simulink library "PV_lib"  (R2016b)
settings: Solver=ode45  StartTime=0.0  StopTime=10.0  RelTol=1e-3  EnableMultiTasking=on
undefined symbols (not defined in the file): C, D, DiscIntNeverNeededParam, f, I_ki, I_kp, Iac_max, Id_at_max, Iq_at_max, L, PLL_Ki, PLL_Kp, PLL_time_step, Roff, Tau, Td_es_min, Tds, Ts, Vdc_max
libraries: powerlib x42, simulink x16, cstextras x4, powerlib_extras x3, Batt_lib x1, powerlib_meascontrol x1
(part 2 of 2)

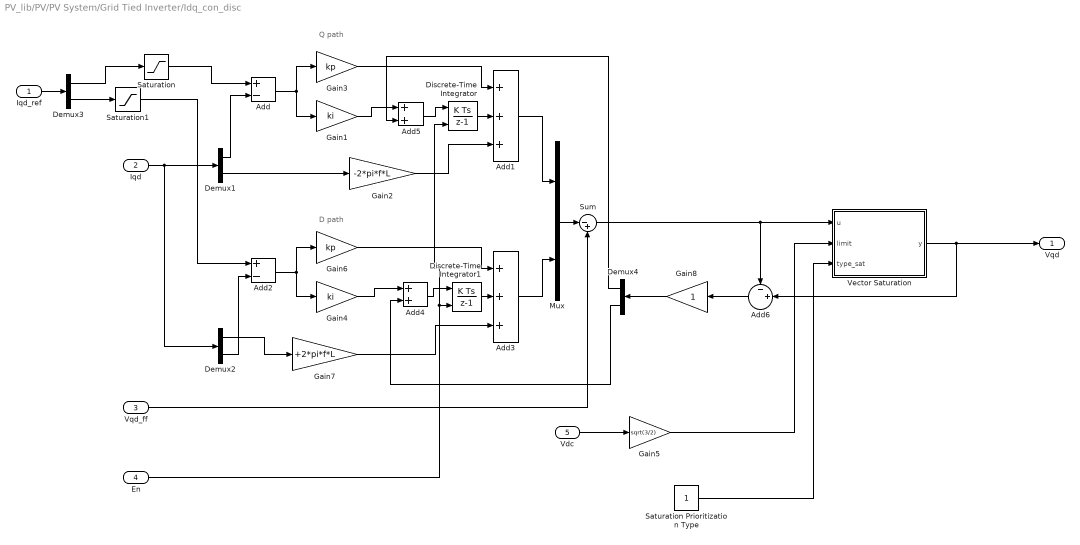
== system PV_lib/PV/PV System/Grid Tied Inverter/Idq_con_disc ==
  note: D path
  note: Q path
  Iqd_ref : Inport
  Iqd : Inport  Port=2
  Vqd_ff : Inport  Port=3  PortDimensions=2
  En : Inport  Port=4  OutDataTypeStr=boolean  PortDimensions=1
  Vdc : Inport  Port=5  PortDimensions=1
  Add : Sum  Inputs=+-
  Add1 : Sum  Inputs=+++
  Add2 : Sum  Inputs=+-
  Add3 : Sum  Inputs=+++
  Add4 : Sum
  Add5 : Sum
  Add6 : Sum  Inputs=-+|
  Demux{1..4} (4 alike) : Demux  Outputs=2
  Discrete-Time Integrator : DiscreteIntegrator  ExternalReset=rising  InitialConditionSetting=Compatibility  SampleTime=Ts  ICPrevOutput=DiscIntNeverNeededParam  ICPrevScaledInput=DiscIntNeverNeededParam
  Discrete-Time Integrator1 : DiscreteIntegrator  ExternalReset=rising  InitialConditionSetting=Compatibility  SampleTime=Ts  ICPrevOutput=DiscIntNeverNeededParam  ICPrevScaledInput=DiscIntNeverNeededParam
  Gain1 : Gain  Gain=ki
  Gain2 : Gain  Gain=-2*pi*f*L
  Gain3 : Gain  Gain=kp
  Gain4 : Gain  Gain=ki
  Gain5 : Gain  Gain=sqrt(3/2)
  Gain6 : Gain  Gain=kp
  Gain7 : Gain  Gain=+2*pi*f*L
  Gain8 : Gain
  Mux : Mux  Inputs=2
  Saturation : Saturate  UpperLimit=iq_max  LowerLimit=-iq_max
  Saturation Prioritization Type : Constant
  Saturation1 : Saturate  UpperLimit=id_max  LowerLimit=-id_max
  Sum : Sum  Inputs=|-+
  Vector Saturation : MATLAB Function  TreatAsAtomicUnit=on
  Vqd : Outport
  wires:
  Vdc/1 -> Gain5/1
  Add6/1 -> Gain8/1
  Gain5/1 -> Vector Saturation/2(limit)
  Saturation Prioritization Type/1 -> Vector Saturation/3(type_sat)
  Vqd_ff/1 -> Sum/2
  Demux2/1 -> Gain7/1
  Demux4/1 -> Add5/2
  Saturation/1 -> Add/1
  Saturation1/1 -> Add2/1
  Iqd_ref/1 -> Demux3/1
  Gain8/1 -> Demux4/1
  Add2/1 -> Gain6/1, Gain4/1
  Demux1/2 -> Gain2/1
  Vector Saturation/1(y) -> Add6/2, Vqd/1
  Demux1/1 -> Add/2
  Gain3/1 -> Add1/1
  Sum/1 -> Add6/1, Vector Saturation/1(u)
  Add1/1 -> Mux/1
  Gain4/1 -> Add4/1
  Add5/1 -> Discrete-Time Integrator/1
  Demux3/1 -> Saturation/1
  Add4/1 -> Discrete-Time Integrator1/1
  Iqd/1 -> Demux1/1, Demux2/1
  Discrete-Time Integrator/1 -> Add1/2
  Demux3/2 -> Saturation1/1
  Gain2/1 -> Add1/3
  Gain1/1 -> Add5/1
  En/1 -> Discrete-Time Integrator1/2, Discrete-Time Integrator/2
  Add3/1 -> Mux/2
  Demux2/2 -> Add2/2
  Gain7/1 -> Add3/3
  Discrete-Time Integrator1/1 -> Add3/2
  Mux/1 -> Sum/1
  Demux4/2 -> Add4/2
  Gain6/1 -> Add3/1
  Add/1 -> Gain3/1, Gain1/1

== system PV_lib/PV/PV System/Grid Tied Inverter/Modulator ==
  Vqd : Inport
  Vdc : Inport  Port=2
  Delay : Delay  DelayLength=1  InitialCondition=[0 0]  SampleTime=Ts
  IC : InitialCondition  Value=Vdc_nom
  Mult1 : Product  Inputs=*/
  Saturation : Saturate  UpperLimit=1  LowerLimit=-1
  dqd : Outport
  wires:
  Mult1/1 -> Saturation/1
  Saturation/1 -> Delay/1
  Vqd/1 -> Mult1/1
  Vdc/1 -> IC/1
  IC/1 -> Mult1/2
  Delay/1 -> dqd/1

== system PV_lib/PV/PV System/Grid Tied Inverter/PLL_disc ==
  note: Theta = 0 at phase A start.
  note: This block should use a normalized to +-1 abc input voltage
  abc : Inport  PortDimensions=3
  Demux1 : Demux  Outputs=2
  Discrete VCO : Subsystem
  Interval Test : simulink/Logic and Bit Operations/Interval Test  IntervalClosedRight=on  uplimit=PLL_lock_window  IntervalClosedLeft=on  lowlimit=-PLL_lock_window  OutDataTypeStr=boolean
  Interval Test1 : simulink/Logic and Bit Operations/Interval Test  IntervalClosedRight=on  uplimit=2*pi*f*(1+PLL_freq_range)  IntervalClosedLeft=on  lowlimit=2*pi*f*(1-PLL_freq_range)  OutDataTypeStr=boolean
  LTI System : Subsystem  BlockChoice=CSS  mask(LTI Block){sys=c2d(tf(1,[1/(f*2*2*pi),1]),Ts), IC=[]}
      mask prompts: sys "LTI system variable"; IC "Initial states (state-space only)"
      mask help:
      | The LTI System block accepts both continuous and discrete LTI models as defined in the Control System Toolbox. Transfer function, state-space, and zero-pole-gain formats are all supported in this block.
      |
      | Note: Initial states are only meaningful for state-space systems.
      mask init:
      | try
      |    % read data to initialize mask variables
      |    [D,Ts,Tdi,Tdo,Tdio,x0,sysname]=...
      |       ltimask('Initialize',gcb,sys,IC);
      |    % update contents
      |    model = bdroot;
      |    df = get_param(model,'dirty');
      |    ltimask('UpdateDiagram',gcb,D,Ts,Tdio);
      |    try      
      |       % Attempt to modify locked library -> error
      |       % Makes block show ??? when loading CSTBLOCKS
      |       % for the first time
      |       set_param(model,'dirty',df)
      |    end
      | catch ME
      |    sys = [];  IC = [];   sysname = '???';
      |    throw(ME)
      | end
      mask Help:
      | The LTI System block accepts any of the three standard LTI models described in the Control System Toolbox: transfer function, zero/pole/gain, or state space. Internally, LTI models will be converted to their state space equivalent for evaluation.
      | <p>
      | In the editable text box labeled <b>LTI System Variable</b>, enter a valid LTI model.
      | <p>
      | In the editable text box labeled <b>Initial States</b> enter the initial state vector.  Initial states are only valid for state-space systems.
      | <p>
      | See also TF, ZPK, SS, LTIMODELS.
      mask Callback sys: ltimask('MaskLTICallback',gcb);
      mask Display: disp(sysname)
  Logical Operator : Logic  AllPortsSameDT=off  OutDataTypeStr=boolean
  PID Controller : simulink/Continuous/PID Controller  Controller=PID  TimeDomain=Discrete-time  SampleTime=Ts  IntegratorMethod=Forward Euler  FilterMethod=Forward Euler  Form=Parallel  UseFilter=on  ControllerParametersSource=internal  P=PLL_Kp  I=PLL_Ki  D=0  N=100  InitialConditionSource=internal  InitialConditionForIntegrator=2*pi*f  InitialConditionForFilter=0  ExternalReset=none  ZeroCross=off  LimitOutput=on  UpperSaturationLimit=2*pi*(f*(1+PLL_freq_range))  LowerSaturationLimit=2*pi*(f*(1-PLL_freq_range))  LinearizeAsGain=on  AntiWindupMode=clamping  Kb=1  TrackingMode=off  Kt=1  PParamMin=[]  PParamMax=[]  IParamMin=[]  IParamMax=[]  DParamMin=[]  DParamMax=[]  NParamMin=[]  NParamMax=[]  KbParamMin=[]  KbParamMax=[]  KtParamMin=[]  KtParamMax=[]  POutMin=[]  POutMax=[]  IOutMin=[]  IOutMax=[]  DOutMin=[]  DOutMax=[]  NOutMin=[]  NOutMax=[]  KbOutMin=[]  KbOutMax=[]  KtOutMin=[]  KtOutMax=[]  IntegratorOutMin=[]  IntegratorOutMax=[]  FilterOutMin=[]  FilterOutMax=[]  SumOutMin=[]  SumOutMax=[]  SumI1OutMin=[]  SumI1OutMax=[]  SumI2OutMin=[]  SumI2OutMax=[]  SumI3OutMin=[]  SumI3OutMax=[]  SumDOutMin=[]  SumDOutMax=[]  SaturationOutMin=[]  SaturationOutMax=[]  IntegratorContinuousStateAttributes=''  IntegratorStateMustResolveToSignalObject=off  IntegratorRTWStateStorageClass=Auto  FilterContinuousStateAttributes=''  FilterStateMustResolveToSignalObject=off  FilterRTWStateStorageClass=Auto  DifferentiatorICPrevScaledInput=0  DifferentiatorOutMin=[]  DifferentiatorOutMax=[]
  Rate Transition : RateTransition  OutPortSampleTime=PLL_time_step
  Subsystem : Subsystem
  Sum : Sum  Inputs=|+-
  Terminator : Terminator
  Terminator1 : Terminator
  Terminator2 : Terminator
  zero : Constant  Value=0
  theta : Outport
  freq : Outport  Port=2
  locked : Outport  Port=3
  wires:
  PID Controller/1 -> freq/1, Discrete VCO/1(In1), Interval Test1/1
  LTI System/1(Out1) -> Interval Test/1
  Demux1/2 -> Terminator2/1  "Vq"
  Demux1/1 -> Sum/1, LTI System/1(In1)  "Vd"
  Discrete VCO/3(theta) -> theta/1, Subsystem/2(theta)
  Logical Operator/1 -> locked/1
  Rate Transition/1 -> Subsystem/1(abc)
  zero/1 -> Sum/2
  Interval Test/1 -> Logical Operator/1
  Interval Test1/1 -> Logical Operator/2
  abc/1 -> Rate Transition/1
  Subsystem/1(qd) -> Demux1/1
  Discrete VCO/1(Cos) -> Terminator/1
  Discrete VCO/2(Sin) -> Terminator1/1
  Sum/1 -> PID Controller/1

== system PV_lib/PV/PV System/Grid Tied Inverter/Subsystem ==
  qd : Inport  OutDataTypeStr=double  PortDimensions=2
  theta : Inport  Port=2  OutDataTypeStr=double  PortDimensions=1
  Mux : Mux  Inputs=3
  Mux1 : Mux  Inputs=2
  qd>a : Fcn  Expr=u[1]*cos(u[3])-u[2]*sin(u[3])
  qd>b : Fcn  Expr=u[1]*cos(u[3]-2*pi/3)-u[2]*sin(u[3]-2*pi/3)
  qd>c : Fcn  Expr=u[1]*cos(u[3]+2*pi/3)-u[2]*sin(u[3]+2*pi/3)
  abc : Outport  OutDataTypeStr=double  PortDimensions=3
  wires:
  qd>a/1 -> Mux/1
  Mux1/1 -> qd>a/1, qd>b/1, qd>c/1
  theta/1 -> Mux1/2
  qd>c/1 -> Mux/3
  qd/1 -> Mux1/1
  qd>b/1 -> Mux/2
  Mux/1 -> abc/1

== system PV_lib/PV/PV System/Grid Tied Inverter/Subsystem1 ==
  abc : Inport  OutDataTypeStr=double  PortDimensions=3
  theta : Inport  Port=2  OutDataTypeStr=double  PortDimensions=1
  Mux : Mux  Inputs=2
  Mux1 : Mux  Inputs=2
  abc>d : Fcn  Expr=2/3*(u[1]*cos(u[4])+u[2]*cos(u[4]-2*pi/3)+u[3]*cos(u[4]+2*pi/3))
  abc>q : Fcn  Expr=2/3*(-u[1]*sin(u[4])-u[2]*sin(u[4]-2*pi/3)-u[3]*sin(u[4]+2*pi/3))
  qd : Outport  OutDataTypeStr=double  PortDimensions=2
  wires:
  abc/1 -> Mux1/1
  theta/1 -> Mux1/2
  abc>q/1 -> Mux/2
  abc>d/1 -> Mux/1
  Mux/1 -> qd/1
  Mux1/1 -> abc>d/1, abc>q/1

== system PV_lib/PV/PV System/Grid Tied Inverter/Windowed Limit ==
  Signal : Inport
  Threshold : Inport  Port=2
  Abs : Abs
  Relational Operator2 : RelationalOperator  Operator=>  OutDataTypeStr=boolean  RndMeth=Nearest
  TestOut : Outport
  wires:
  Signal/1 -> Abs/1
  Threshold/1 -> Relational Operator2/2
  Relational Operator2/1 -> TestOut/1
  Abs/1 -> Relational Operator2/1

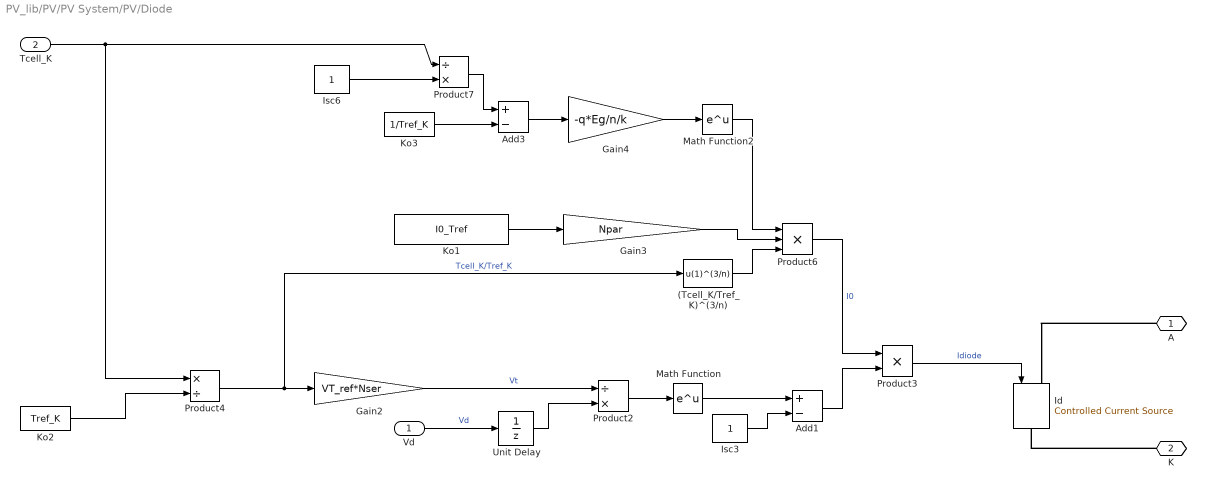
== system PV_lib/PV/PV System/PV/Diode ==
  Vd : Inport
  Tcell_K : Inport  Port=2
  (Tcell_K/Tref_K)^(3/n) : Fcn  Expr=u(1)^(3/n)
  Add1 : Sum  Inputs=+-
  Add3 : Sum  Inputs=+-
  Gain2 : Gain  Gain=VT_ref*Nser
  Gain3 : Gain  Gain=Npar
  Gain4 : Gain  Gain=-q*Eg/n/k
  Id : powerlib/Electrical Sources/Controlled Current Source  Initialize=on  Source_Type=AC  Amplitude=0  Phase=0  Frequency=0  Measurements=None
  Isc3 : Constant
  Isc6 : Constant
  Ko1 : Constant  Value=I0_Tref
  Ko2 : Constant  Value=Tref_K
  Ko3 : Constant  Value=1/Tref_K
  Math Function : Math  SaturateOnIntegerOverflow=on
  Math Function2 : Math  SaturateOnIntegerOverflow=on
  Product2 : Product  Inputs=/*  RndMeth=Zero
  Product3 : Product  RndMeth=Zero
  Product4 : Product  Inputs=*/  RndMeth=Zero
  Product6 : Product  Inputs=3  RndMeth=Zero
  Product7 : Product  Inputs=/*  RndMeth=Zero
  Unit Delay : UnitDelay  SampleTime=Ts
  A : PMIOPort  Port=1  Side=Left
  K : PMIOPort  Port=2  Side=Right
  wires:
  Vd/1 -> Unit Delay/1  "Vd"
  Gain2/1 -> Product2/1  "Vt"
  Product2/1 -> Math Function/1
  Math Function/1 -> Add1/1
  Isc3/1 -> Add1/2
  Add1/1 -> Product3/2
  Product3/1 -> Id/1  "Idiode"
  Ko2/1 -> Product4/2
  Product4/1 -> Gain2/1, (Tcell_K/Tref_K)^(3/n)/1  "Tcell_K/Tref_K"
  Ko1/1 -> Gain3/1
  Ko3/1 -> Add3/2
  Isc6/1 -> Product7/2
  Tcell_K/1 -> Product4/1, Product7/1
  Product7/1 -> Add3/1
  Add3/1 -> Gain4/1
  Gain4/1 -> Math Function2/1
  (Tcell_K/Tref_K)^(3/n)/1 -> Product6/3
  Gain3/1 -> Product6/2
  Math Function2/1 -> Product6/1
  Product6/1 -> Product3/1  "I0"
  Unit Delay/1 -> Product2/2
  connections:
  A/RConn1 -- Id/LConn1
  K/RConn1 -- Id/RConn1

== system PV_lib/PV/PV System/PV/Light current IL ==
  Temperature : Inport
  Irradiance : Inport  Port=2
  Gain : Gain  Gain=K0
  Gain2 : Gain  Gain=Isc_Tref
  Gain3 : Gain  Gain=Npar/Gnom
  Ko1 : Constant  Value=273.15
  Ko2 : Constant  Value=Tref_K
  Ko3 : Constant
  Product3 : Product  RndMeth=Zero
  Sum3 : Sum  SaturateOnIntegerOverflow=on  InputSameDT=on  OutDataTypeStr=Inherit: Same as first input
  Sum4 : Sum  Inputs=+-  SaturateOnIntegerOverflow=on  InputSameDT=on  OutDataTypeStr=Inherit: Same as first input
  Sum5 : Sum  SaturateOnIntegerOverflow=on  InputSameDT=on  OutDataTypeStr=Inherit: Same as first input
  IL : Outport
  Tcell_K : Outport  Port=2
  wires:
  Ko1/1 -> Sum3/2
  Sum3/1 -> Tcell_K/1, Sum4/1
  Ko2/1 -> Sum4/2
  Sum4/1 -> Gain/1
  Gain/1 -> Sum5/1
  Ko3/1 -> Sum5/2
  Sum5/1 -> Gain2/1
  Gain2/1 -> Product3/1
  Product3/1 -> Gain3/1
  Temperature/1 -> Sum3/1
  Gain3/1 -> IL/1
  Irradiance/1 -> Product3/2

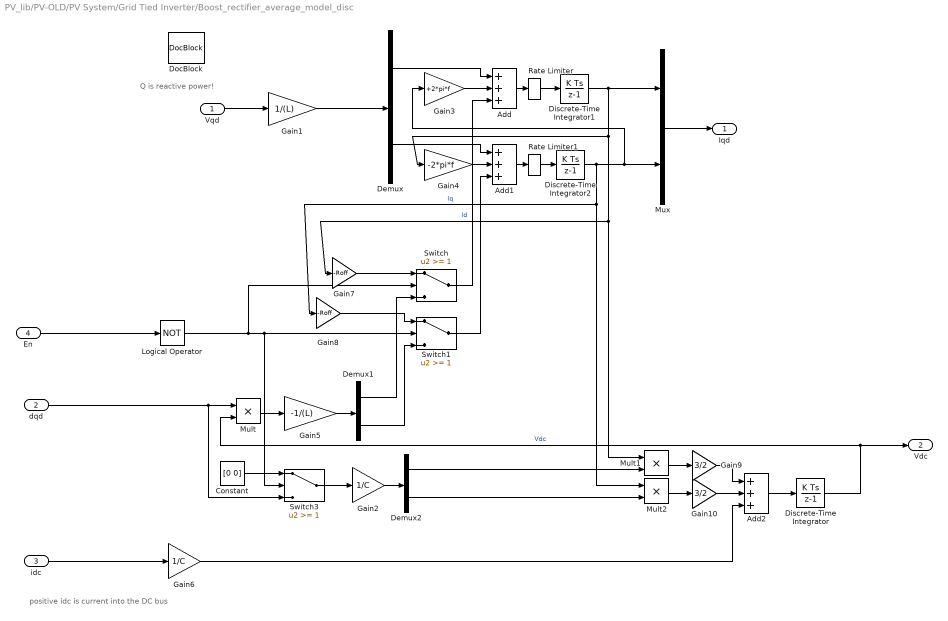
== system PV_lib/PV-OLD/PV System/Grid Tied Inverter/Boost_rectifier_average_model_disc ==
  note: Q is reactive power!
  note: positive idc is current into the DC bus
  Vqd : Inport
  dqd : Inport  Port=2  PortDimensions=2
  idc : Inport  Port=3
  En : Inport  Port=4  OutDataTypeStr=boolean
  Add : Sum  Inputs=+++
  Add1 : Sum  Inputs=+++
  Add2 : Sum  Inputs=+++
  Constant : Constant  Value=[0 0]
  Demux : Demux  Outputs=2
  Demux1 : Demux  Outputs=2
  Demux2 : Demux  Outputs=2
  Discrete-Time Integrator : DiscreteIntegrator  InitialCondition=Vdc_nom  InitialConditionSetting=Compatibility  SampleTime=Tds  ICPrevOutput=DiscIntNeverNeededParam  ICPrevScaledInput=DiscIntNeverNeededParam
  Discrete-Time Integrator1 : DiscreteIntegrator  InitialConditionSetting=Compatibility  SampleTime=Tds  ICPrevOutput=DiscIntNeverNeededParam  ICPrevScaledInput=DiscIntNeverNeededParam
  Discrete-Time Integrator2 : DiscreteIntegrator  InitialConditionSetting=Compatibility  SampleTime=Tds  ICPrevOutput=DiscIntNeverNeededParam  ICPrevScaledInput=DiscIntNeverNeededParam
  DocBlock : simulink/Model-Wide Utilities/DocBlock  DocumentType=Text
      content=|
      | Model is based on average boost rectifier model.
      |
      | Enable signal switches in a large resistor in place of the average IGBT voltage.
      | Also, it zero's currents going into DC bus voltage equation since there was some leakage there.
      |
      | The clamping of diodes at IGBT turn-off is not modeled here!
  Gain1 : Gain  Gain=1/(L)
  Gain10 : Gain  Gain=3/2
  Gain2 : Gain  Gain=1/C
  Gain3 : Gain  Gain=+2*pi*f
  Gain4 : Gain  Gain=-2*pi*f
  Gain5 : Gain  Gain=-1/(L)
  Gain6 : Gain  Gain=1/C
  Gain7 : Gain  Gain=-Roff
  Gain8 : Gain  Gain=-Roff
  Gain9 : Gain  Gain=3/2
  Logical Operator : Logic  Operator=NOT  AllPortsSameDT=off  OutDataTypeStr=boolean
  Mult : Product  Inputs=**
  Mult1 : Product  Inputs=**
  Mult2 : Product  Inputs=**
  Mux : Mux  Inputs=2
  Rate Limiter : RateLimiter  RisingSlewLimit=1e6  FallingSlewLimit=-1e6  SampleTimeMode=inherited
  Rate Limiter1 : RateLimiter  RisingSlewLimit=1e6  FallingSlewLimit=-1e6  SampleTimeMode=inherited
  Switch : Switch  Threshold=1
  Switch1 : Switch  Threshold=1
  Switch3 : Switch  Threshold=1
  Iqd : Outport
  Vdc : Outport  Port=2
  wires:
  Rate Limiter1/1 -> Discrete-Time Integrator2/1
  Rate Limiter/1 -> Discrete-Time Integrator1/1
  Add1/1 -> Rate Limiter1/1
  dqd/1 -> Mult/1, Switch3/3
  Gain8/1 -> Switch1/1
  Discrete-Time Integrator2/1 -> Mux/2, Gain3/1, Mult2/1, Gain8/1  "Iq"
  Demux1/2 -> Switch1/3
  Mult1/1 -> Gain9/1
  Switch1/1 -> Add1/3
  Add/1 -> Rate Limiter/1
  Switch/1 -> Add/3
  Gain1/1 -> Demux/1
  Gain5/1 -> Demux1/1
  Mult2/1 -> Gain10/1
  Constant/1 -> Switch3/1
  Gain9/1 -> Add2/1
  Demux2/2 -> Mult2/2
  idc/1 -> Gain6/1
  Mult/1 -> Gain5/1
  Add2/1 -> Discrete-Time Integrator/1
  Gain7/1 -> Switch/1
  Demux/1 -> Add/1
  En/1 -> Logical Operator/1
  Discrete-Time Integrator1/1 -> Mux/1, Gain4/1, Mult1/1, Gain7/1  "Id"
  Mux/1 -> Iqd/1
  Switch3/1 -> Gain2/1
  Logical Operator/1 -> Switch/2, Switch1/2, Switch3/2
  Gain10/1 -> Add2/2
  Gain6/1 -> Add2/3
  Gain2/1 -> Demux2/1
  Demux1/1 -> Switch/3
  Vqd/1 -> Gain1/1
  Gain4/1 -> Add1/2
  Gain3/1 -> Add/2
  Demux2/1 -> Mult1/2
  Demux/2 -> Add1/1
  Discrete-Time Integrator/1 -> Vdc/1, Mult/2  "Vdc"

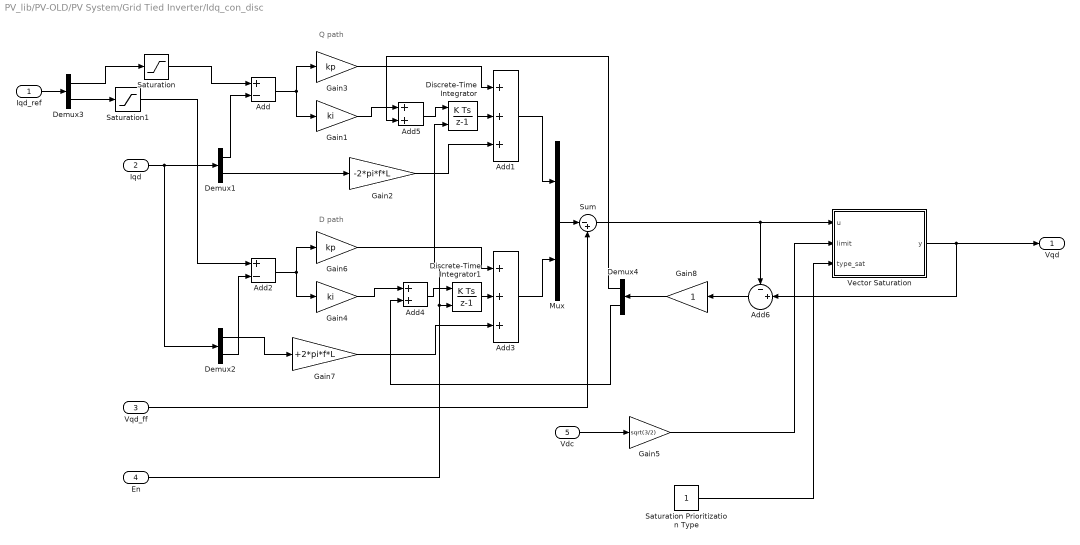
== system PV_lib/PV-OLD/PV System/Grid Tied Inverter/Idq_con_disc ==
  note: Q path
  note: D path
  Iqd_ref : Inport
  Iqd : Inport  Port=2
  Vqd_ff : Inport  Port=3  PortDimensions=2
  En : Inport  Port=4  OutDataTypeStr=boolean  PortDimensions=1
  Vdc : Inport  Port=5  PortDimensions=1
  Add : Sum  Inputs=+-
  Add1 : Sum  Inputs=+++
  Add2 : Sum  Inputs=+-
  Add3 : Sum  Inputs=+++
  Add4 : Sum
  Add5 : Sum
  Add6 : Sum  Inputs=-+|
  Demux{1..4} (4 alike) : Demux  Outputs=2
  Discrete-Time Integrator : DiscreteIntegrator  ExternalReset=rising  InitialConditionSetting=Compatibility  SampleTime=Td_es_min  ICPrevOutput=DiscIntNeverNeededParam  ICPrevScaledInput=DiscIntNeverNeededParam
  Discrete-Time Integrator1 : DiscreteIntegrator  ExternalReset=rising  InitialConditionSetting=Compatibility  SampleTime=Td_es_min  ICPrevOutput=DiscIntNeverNeededParam  ICPrevScaledInput=DiscIntNeverNeededParam
  Gain1 : Gain  Gain=ki
  Gain2 : Gain  Gain=-2*pi*f*L
  Gain3 : Gain  Gain=kp
  Gain4 : Gain  Gain=ki
  Gain5 : Gain  Gain=sqrt(3/2)
  Gain6 : Gain  Gain=kp
  Gain7 : Gain  Gain=+2*pi*f*L
  Gain8 : Gain
  Mux : Mux  Inputs=2
  Saturation : Saturate  UpperLimit=iq_max  LowerLimit=-iq_max
  Saturation Prioritization Type : Constant
  Saturation1 : Saturate  UpperLimit=id_max  LowerLimit=-id_max
  Sum : Sum  Inputs=|-+
  Vector Saturation : MATLAB Function  TreatAsAtomicUnit=on
  Vqd : Outport
  wires:
  Add/1 -> Gain1/1, Gain3/1
  Gain6/1 -> Add3/1
  Demux4/2 -> Add4/2
  Mux/1 -> Sum/1
  Discrete-Time Integrator1/1 -> Add3/2
  Gain7/1 -> Add3/3
  Demux2/2 -> Add2/2
  Add3/1 -> Mux/2
  En/1 -> Discrete-Time Integrator/2, Discrete-Time Integrator1/2
  Gain1/1 -> Add5/1
  Gain2/1 -> Add1/3
  Demux3/2 -> Saturation1/1
  Discrete-Time Integrator/1 -> Add1/2
  Iqd/1 -> Demux2/1, Demux1/1
  Add4/1 -> Discrete-Time Integrator1/1
  Demux3/1 -> Saturation/1
  Add5/1 -> Discrete-Time Integrator/1
  Gain4/1 -> Add4/1
  Add1/1 -> Mux/1
  Sum/1 -> Vector Saturation/1(u), Add6/1
  Gain3/1 -> Add1/1
  Demux1/1 -> Add/2
  Vector Saturation/1(y) -> Vqd/1, Add6/2
  Demux1/2 -> Gain2/1
  Add2/1 -> Gain4/1, Gain6/1
  Gain8/1 -> Demux4/1
  Iqd_ref/1 -> Demux3/1
  Saturation1/1 -> Add2/1
  Saturation/1 -> Add/1
  Demux4/1 -> Add5/2
  Demux2/1 -> Gain7/1
  Vqd_ff/1 -> Sum/2
  Saturation Prioritization Type/1 -> Vector Saturation/3(type_sat)
  Gain5/1 -> Vector Saturation/2(limit)
  Add6/1 -> Gain8/1
  Vdc/1 -> Gain5/1

== system PV_lib/PV-OLD/PV System/Grid Tied Inverter/Modulator ==
  Vqd : Inport
  Vdc : Inport  Port=2
  Delay : Delay  DelayLength=1  InitialCondition=[0 0]  SampleTime=Td_es_min
  IC : InitialCondition  Value=Vdc_nom
  Mult1 : Product  Inputs=*/
  Saturation : Saturate  UpperLimit=1  LowerLimit=-1
  dqd : Outport
  wires:
  Delay/1 -> dqd/1
  IC/1 -> Mult1/2
  Vdc/1 -> IC/1
  Vqd/1 -> Mult1/1
  Saturation/1 -> Delay/1
  Mult1/1 -> Saturation/1

== system PV_lib/PV-OLD/PV System/Grid Tied Inverter/PLL_disc ==
  note: This block should use a normalized to +-1 abc input voltage
  note: Theta = 0 at phase A start.
  abc : Inport  PortDimensions=3
  Demux1 : Demux  Outputs=2
  Discrete VCO : Subsystem
  Interval Test : simulink/Logic and Bit Operations/Interval Test  IntervalClosedRight=on  uplimit=PLL_lock_window  IntervalClosedLeft=on  lowlimit=-PLL_lock_window  OutDataTypeStr=boolean
  Interval Test1 : simulink/Logic and Bit Operations/Interval Test  IntervalClosedRight=on  uplimit=2*pi*f*(1+PLL_freq_range)  IntervalClosedLeft=on  lowlimit=2*pi*f*(1-PLL_freq_range)  OutDataTypeStr=boolean
  LTI System : Subsystem  BlockChoice=CSS  mask(LTI Block){sys=c2d(tf(1,[1/(f*2*2*pi),1]),Td_es_min), IC=[]}
      mask prompts: sys "LTI system variable"; IC "Initial states (state-space only)"
      mask help:
      | The LTI System block accepts both continuous and discrete LTI models as defined in the Control System Toolbox. Transfer function, state-space, and zero-pole-gain formats are all supported in this block.
      |
      | Note: Initial states are only meaningful for state-space systems.
      mask init: same as PV_lib/PV/PV System/Grid Tied Inverter/PLL_disc/LTI System
      mask Help:
      | The LTI System block accepts any of the three standard LTI models described in the Control System Toolbox: transfer function, zero/pole/gain, or state space. Internally, LTI models will be converted to their state space equivalent for evaluation.
      | <p>
      | In the editable text box labeled <b>LTI System Variable</b>, enter a valid LTI model.
      | <p>
      | In the editable text box labeled <b>Initial States</b> enter the initial state vector.  Initial states are only valid for state-space systems.
      | <p>
      | See also TF, ZPK, SS, LTIMODELS.
      mask Callback sys: ltimask('MaskLTICallback',gcb);
      mask Display: disp(sysname)
  Logical Operator : Logic  AllPortsSameDT=off  OutDataTypeStr=boolean
  PID Controller : simulink/Continuous/PID Controller  Controller=PID  TimeDomain=Discrete-time  SampleTime=PLL_time_step  IntegratorMethod=Forward Euler  FilterMethod=Forward Euler  Form=Parallel  UseFilter=on  ControllerParametersSource=internal  P=PLL_Kp  I=PLL_Ki  D=0  N=100  InitialConditionSource=internal  InitialConditionForIntegrator=2*pi*f  InitialConditionForFilter=0  ExternalReset=none  ZeroCross=off  LimitOutput=on  UpperSaturationLimit=2*pi*(f*(1+PLL_freq_range))  LowerSaturationLimit=2*pi*(f*(1-PLL_freq_range))  LinearizeAsGain=on  AntiWindupMode=clamping  Kb=1  TrackingMode=off  Kt=1  PParamMin=[]  PParamMax=[]  IParamMin=[]  IParamMax=[]  DParamMin=[]  DParamMax=[]  NParamMin=[]  NParamMax=[]  KbParamMin=[]  KbParamMax=[]  KtParamMin=[]  KtParamMax=[]  POutMin=[]  POutMax=[]  IOutMin=[]  IOutMax=[]  DOutMin=[]  DOutMax=[]  NOutMin=[]  NOutMax=[]  KbOutMin=[]  KbOutMax=[]  KtOutMin=[]  KtOutMax=[]  IntegratorOutMin=[]  IntegratorOutMax=[]  FilterOutMin=[]  FilterOutMax=[]  SumOutMin=[]  SumOutMax=[]  SumI1OutMin=[]  SumI1OutMax=[]  SumI2OutMin=[]  SumI2OutMax=[]  SumI3OutMin=[]  SumI3OutMax=[]  SumDOutMin=[]  SumDOutMax=[]  SaturationOutMin=[]  SaturationOutMax=[]  IntegratorContinuousStateAttributes=''  IntegratorStateMustResolveToSignalObject=off  IntegratorRTWStateStorageClass=Auto  FilterContinuousStateAttributes=''  FilterStateMustResolveToSignalObject=off  FilterRTWStateStorageClass=Auto  DifferentiatorICPrevScaledInput=0  DifferentiatorOutMin=[]  DifferentiatorOutMax=[]
  Rate Transition : RateTransition  OutPortSampleTime=PLL_time_step
  Subsystem : Subsystem
  Sum : Sum  Inputs=|+-
  Terminator : Terminator
  Terminator1 : Terminator
  Terminator2 : Terminator
  zero : Constant  Value=0
  theta : Outport
  freq : Outport  Port=2
  locked : Outport  Port=3
  wires:
  Sum/1 -> PID Controller/1
  Discrete VCO/2(Sin) -> Terminator1/1
  Discrete VCO/1(Cos) -> Terminator/1
  Subsystem/1(qd) -> Demux1/1
  abc/1 -> Rate Transition/1
  Interval Test1/1 -> Logical Operator/2
  Interval Test/1 -> Logical Operator/1
  zero/1 -> Sum/2
  Rate Transition/1 -> Subsystem/1(abc)
  Logical Operator/1 -> locked/1
  Discrete VCO/3(theta) -> Subsystem/2(theta), theta/1
  Demux1/1 -> LTI System/1(In1), Sum/1  "Vd"
  Demux1/2 -> Terminator2/1  "Vq"
  LTI System/1(Out1) -> Interval Test/1
  PID Controller/1 -> Interval Test1/1, Discrete VCO/1(In1), freq/1

== system PV_lib/PV-OLD/PV System/Grid Tied Inverter/RMS_Calculator ==
  Signal : Inport
  Discrete Mean value6 : powerlib_extras/Discrete Measurements/Discrete  Mean value  Freq=60/4  Vinit=0  Ts=Ts
  Memory : Memory
  Product3 : Product  RndMeth=Zero
  Signed Sqrt : Sqrt  SaturateOnIntegerOverflow=on
  RMS_Signal : Outport
  wires:
  Memory/1 -> Discrete Mean value6/1
  Signed Sqrt/1 -> RMS_Signal/1
  Discrete Mean value6/1 -> Signed Sqrt/1
  Product3/1 -> Memory/1
  Signal/1 -> Product3/2, Product3/1

== system PV_lib/PV-OLD/PV System/Grid Tied Inverter/Subsystem ==
  qd : Inport  OutDataTypeStr=double  PortDimensions=2
  theta : Inport  Port=2  OutDataTypeStr=double  PortDimensions=1
  Mux : Mux  Inputs=3
  Mux1 : Mux  Inputs=2
  qd>a : Fcn  Expr=u[1]*cos(u[3])-u[2]*sin(u[3])
  qd>b : Fcn  Expr=u[1]*cos(u[3]-2*pi/3)-u[2]*sin(u[3]-2*pi/3)
  qd>c : Fcn  Expr=u[1]*cos(u[3]+2*pi/3)-u[2]*sin(u[3]+2*pi/3)
  abc : Outport  OutDataTypeStr=double  PortDimensions=3
  wires:
  Mux/1 -> abc/1
  qd>b/1 -> Mux/2
  qd/1 -> Mux1/1
  qd>c/1 -> Mux/3
  theta/1 -> Mux1/2
  Mux1/1 -> qd>c/1, qd>b/1, qd>a/1
  qd>a/1 -> Mux/1

== system PV_lib/PV-OLD/PV System/Grid Tied Inverter/Subsystem1 ==
  abc : Inport  OutDataTypeStr=double  PortDimensions=3
  theta : Inport  Port=2  OutDataTypeStr=double  PortDimensions=1
  Mux : Mux  Inputs=2
  Mux1 : Mux  Inputs=2
  abc>d : Fcn  Expr=2/3*(u[1]*cos(u[4])+u[2]*cos(u[4]-2*pi/3)+u[3]*cos(u[4]+2*pi/3))
  abc>q : Fcn  Expr=2/3*(-u[1]*sin(u[4])-u[2]*sin(u[4]-2*pi/3)-u[3]*sin(u[4]+2*pi/3))
  qd : Outport  OutDataTypeStr=double  PortDimensions=2
  wires:
  Mux1/1 -> abc>q/1, abc>d/1
  Mux/1 -> qd/1
  abc>d/1 -> Mux/1
  abc>q/1 -> Mux/2
  theta/1 -> Mux1/2
  abc/1 -> Mux1/1

== system PV_lib/PV-OLD/PV System/Grid Tied Inverter/Windowed Limit ==
  Signal : Inport
  Threshold : Inport  Port=2
  Abs : Abs
  Relational Operator2 : RelationalOperator  Operator=>  OutDataTypeStr=boolean  RndMeth=Nearest
  TestOut : Outport
  wires:
  Abs/1 -> Relational Operator2/1
  Relational Operator2/1 -> TestOut/1
  Threshold/1 -> Relational Operator2/2
  Signal/1 -> Abs/1

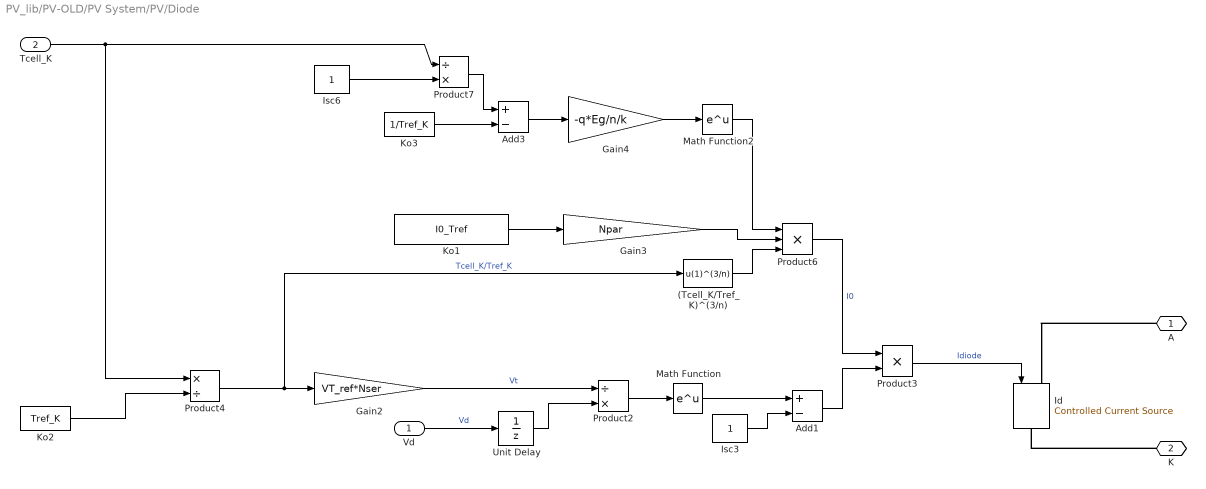
== system PV_lib/PV-OLD/PV System/PV/Diode ==
  Vd : Inport
  Tcell_K : Inport  Port=2
  (Tcell_K/Tref_K)^(3/n) : Fcn  Expr=u(1)^(3/n)
  Add1 : Sum  Inputs=+-
  Add3 : Sum  Inputs=+-
  Gain2 : Gain  Gain=VT_ref*Nser
  Gain3 : Gain  Gain=Npar
  Gain4 : Gain  Gain=-q*Eg/n/k
  Id : powerlib/Electrical Sources/Controlled Current Source  Initialize=on  Source_Type=AC  Amplitude=0  Phase=0  Frequency=0  Measurements=None
  Isc3 : Constant
  Isc6 : Constant
  Ko1 : Constant  Value=I0_Tref
  Ko2 : Constant  Value=Tref_K
  Ko3 : Constant  Value=1/Tref_K
  Math Function : Math  SaturateOnIntegerOverflow=on
  Math Function2 : Math  SaturateOnIntegerOverflow=on
  Product2 : Product  Inputs=/*  RndMeth=Zero
  Product3 : Product  RndMeth=Zero
  Product4 : Product  Inputs=*/  RndMeth=Zero
  Product6 : Product  Inputs=3  RndMeth=Zero
  Product7 : Product  Inputs=/*  RndMeth=Zero
  Unit Delay : UnitDelay  SampleTime=Ts
  A : PMIOPort  Port=1  Side=Left
  K : PMIOPort  Port=2  Side=Right
  wires:
  Unit Delay/1 -> Product2/2
  Product6/1 -> Product3/1  "I0"
  Math Function2/1 -> Product6/1
  Gain3/1 -> Product6/2
  (Tcell_K/Tref_K)^(3/n)/1 -> Product6/3
  Gain4/1 -> Math Function2/1
  Add3/1 -> Gain4/1
  Product7/1 -> Add3/1
  Tcell_K/1 -> Product7/1, Product4/1
  Isc6/1 -> Product7/2
  Ko3/1 -> Add3/2
  Ko1/1 -> Gain3/1
  Product4/1 -> (Tcell_K/Tref_K)^(3/n)/1, Gain2/1  "Tcell_K/Tref_K"
  Ko2/1 -> Product4/2
  Product3/1 -> Id/1  "Idiode"
  Add1/1 -> Product3/2
  Isc3/1 -> Add1/2
  Math Function/1 -> Add1/1
  Product2/1 -> Math Function/1
  Gain2/1 -> Product2/1  "Vt"
  Vd/1 -> Unit Delay/1  "Vd"
  connections:
  K/RConn1 -- Id/RConn1
  A/RConn1 -- Id/LConn1

== system PV_lib/PV-OLD/PV System/PV/Light current IL ==
  Temperature : Inport
  Irradiance : Inport  Port=2
  Gain : Gain  Gain=K0
  Gain2 : Gain  Gain=Isc_Tref
  Gain3 : Gain  Gain=Npar/Gnom
  Ko1 : Constant  Value=273.15
  Ko2 : Constant  Value=Tref_K
  Ko3 : Constant
  Product3 : Product  RndMeth=Zero
  Sum3 : Sum  SaturateOnIntegerOverflow=on  InputSameDT=on  OutDataTypeStr=Inherit: Same as first input
  Sum4 : Sum  Inputs=+-  SaturateOnIntegerOverflow=on  InputSameDT=on  OutDataTypeStr=Inherit: Same as first input
  Sum5 : Sum  SaturateOnIntegerOverflow=on  InputSameDT=on  OutDataTypeStr=Inherit: Same as first input
  IL : Outport
  Tcell_K : Outport  Port=2
  wires:
  Irradiance/1 -> Product3/2
  Gain3/1 -> IL/1
  Temperature/1 -> Sum3/1
  Product3/1 -> Gain3/1
  Gain2/1 -> Product3/1
  Sum5/1 -> Gain2/1
  Ko3/1 -> Sum5/2
  Gain/1 -> Sum5/1
  Sum4/1 -> Gain/1
  Ko2/1 -> Sum4/2
  Sum3/1 -> Sum4/1, Tcell_K/1
  Ko1/1 -> Sum3/2

== system PV_lib/PV/PV System/Grid Tied Inverter/PLL_disc/Discrete VCO ==
  note: VCO
  In1 : Inport
  Constant : Constant  Value=2*pi
  Discrete-Time Integrator : DiscreteIntegrator  InitialConditionSetting=Compatibility  SampleTime=Ts  ICPrevOutput=DiscIntNeverNeededParam  ICPrevScaledInput=DiscIntNeverNeededParam
  Gain1 : Gain  OutDataTypeStr=double
  Math Function : Math  Operator=mod  SaturateOnIntegerOverflow=on
  Scope2 : Scope
  cos1 : Trigonometry  Operator=cos
  sin1 : Trigonometry
  Cos : Outport
  Sin : Outport  Port=2
  theta : Outport  Port=3
  wires:
  Math Function/1 -> sin1/1, cos1/1, theta/1, Scope2/1
  Discrete-Time Integrator/1 -> Math Function/1
  Gain1/1 -> Discrete-Time Integrator/1
  Constant/1 -> Math Function/2
  sin1/1 -> Sin/1
  cos1/1 -> Cos/1
  In1/1 -> Gain1/1

== system PV_lib/PV/PV System/Grid Tied Inverter/PLL_disc/LTI System ==
  In1 : Inport
  IO Delay : cstextras/Integer Delay (masked)  Td=Tdio  u0=0  Ts=Ts
  Input Delay : cstextras/Integer Delay (masked)  Td=Tdi  u0=0  Ts=Ts
  Internal : DiscreteStateSpace  A=D.a  B=D.b  C=D.c  D=D.d  SampleTime=Ts
  Output Delay : cstextras/Integer Delay (masked)  Td=Tdo  u0=0  Ts=Ts
  Out1 : Outport  InitialOutput=0
  wires:
  In1/1 -> Input Delay/1
  Output Delay/1 -> Out1/1
  Input Delay/1 -> Internal/1
  Internal/1 -> IO Delay/1
  IO Delay/1 -> Output Delay/1

== system PV_lib/PV/PV System/Grid Tied Inverter/PLL_disc/Subsystem ==
  abc : Inport  OutDataTypeStr=double  PortDimensions=3
  theta : Inport  Port=2  OutDataTypeStr=double  PortDimensions=1
  Mux : Mux  Inputs=2
  Mux1 : Mux  Inputs=2
  abc>d : Fcn  Expr=2/3*(u[1]*cos(u[4])+u[2]*cos(u[4]-2*pi/3)+u[3]*cos(u[4]+2*pi/3))
  abc>q : Fcn  Expr=2/3*(-u[1]*sin(u[4])-u[2]*sin(u[4]-2*pi/3)-u[3]*sin(u[4]+2*pi/3))
  qd : Outport  OutDataTypeStr=double  PortDimensions=2
  wires:
  Mux1/1 -> abc>q/1, abc>d/1
  Mux/1 -> qd/1
  abc>d/1 -> Mux/1
  abc>q/1 -> Mux/2
  theta/1 -> Mux1/2
  abc/1 -> Mux1/1

== system PV_lib/PV-OLD/PV System/Grid Tied Inverter/PLL_disc/Discrete VCO ==
  note: VCO
  In1 : Inport
  Constant : Constant  Value=2*pi
  Discrete-Time Integrator : DiscreteIntegrator  InitialConditionSetting=Compatibility  SampleTime=Td_es_min  ICPrevOutput=DiscIntNeverNeededParam  ICPrevScaledInput=DiscIntNeverNeededParam
  Gain1 : Gain  OutDataTypeStr=double
  Math Function : Math  Operator=mod  SaturateOnIntegerOverflow=on
  Scope2 : Scope
  cos1 : Trigonometry  Operator=cos
  sin1 : Trigonometry
  Cos : Outport
  Sin : Outport  Port=2
  theta : Outport  Port=3
  wires:
  In1/1 -> Gain1/1
  cos1/1 -> Cos/1
  sin1/1 -> Sin/1
  Constant/1 -> Math Function/2
  Gain1/1 -> Discrete-Time Integrator/1
  Discrete-Time Integrator/1 -> Math Function/1
  Math Function/1 -> Scope2/1, theta/1, cos1/1, sin1/1

== system PV_lib/PV-OLD/PV System/Grid Tied Inverter/PLL_disc/LTI System ==
  In1 : Inport
  Output Delay : cstextras/Integer Delay (masked)  Td=Tdo  u0=0  Ts=Ts
  Out1 : Outport  InitialOutput=0
  wires:
  ? -> Output Delay/1
  ? -> ?
  ? -> ?
  Output Delay/1 -> Out1/1
  In1/1 -> ?

== system PV_lib/PV-OLD/PV System/Grid Tied Inverter/PLL_disc/Subsystem ==
  abc : Inport  OutDataTypeStr=double  PortDimensions=3
  theta : Inport  Port=2  OutDataTypeStr=double  PortDimensions=1
  Mux : Mux  Inputs=2
  Mux1 : Mux  Inputs=2
  abc>d : Fcn  Expr=2/3*(u[1]*cos(u[4])+u[2]*cos(u[4]-2*pi/3)+u[3]*cos(u[4]+2*pi/3))
  abc>q : Fcn  Expr=2/3*(-u[1]*sin(u[4])-u[2]*sin(u[4]-2*pi/3)-u[3]*sin(u[4]+2*pi/3))
  qd : Outport  OutDataTypeStr=double  PortDimensions=2
  wires:
  abc/1 -> Mux1/1
  theta/1 -> Mux1/2
  abc>q/1 -> Mux/2
  abc>d/1 -> Mux/1
  Mux/1 -> qd/1
  Mux1/1 -> abc>d/1, abc>q/1

== matlab function PV_lib/PV/PV System/Grid Tied Inverter/Idq_con_disc/Vector Saturation ==
  data: u input; y output; limit input; type_sat input
function y = fcn(u, limit, type_sat)
% When the magnitude is of u is greater than limit prioritize the
% saturation to u(type_sat) dimension.  u is two dimensional input.
%#codegen
y=zeros(2,1); % required initialization
u_sign=sign(u);

if(abs(u(1)) > limit)
    u(1) = u_sign(1).*limit;
end
if(abs(u(2)) > limit)
    u(2) =  u_sign(2).*limit;
end
if(u(1)^2 + u(2)^2 > limit^2)
    if(type_sat == 1) % priority given to u(1)
        y(1) = u(1);
        y(2) = u_sign(2) .* sqrt(limit^2 - u(1)^2); 
    else  % priority given to u(2)
        y(2) = u(2);
        y(1) =  u_sign(1) .* sqrt(limit^2 - u(2)^2); 
    end
else
    y = u;
end

== matlab function PV_lib/PV-OLD/PV System/Grid Tied Inverter/Idq_con_disc/Vector Saturation ==
  data: u input; y output; limit input; type_sat input
function y = fcn(u, limit, type_sat)
% When the magnitude is of u is greater than limit prioritize the
% saturation to u(type_sat) dimension.  u is two dimensional input.
%#codegen
y=zeros(2,1); % required initialization
u_sign=sign(u);

if(abs(u(1)) > limit)
    u(1) = u_sign(1).*limit;
end
if(abs(u(2)) > limit)
    u(2) =  u_sign(2).*limit;
end
if(u(1)^2 + u(2)^2 > limit^2)
    if(type_sat == 1) % priority given to u(1)
        y(1) = u(1);
        y(2) = u_sign(2) .* sqrt(limit^2 - u(1)^2); 
    else  % priority given to u(2)
        y(2) = u(2);
        y(1) =  u_sign(1) .* sqrt(limit^2 - u(2)^2); 
    end
else
    y = u;
end
